simulink model "Diagrama2"  (R2023b)
settings: Solver=VariableStepAuto  StartTime=0.0  StopTime=10.0  RelTol=1e-3
settings Model: Creator=Roberd  LastModifiedBy=Roberd

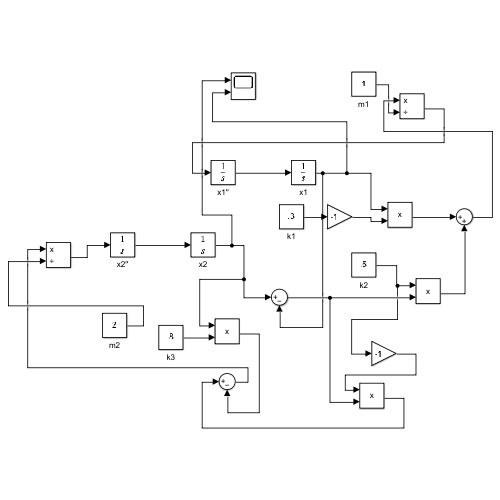
[thumbnail: Simulink's stored preview of the top-level diagram]
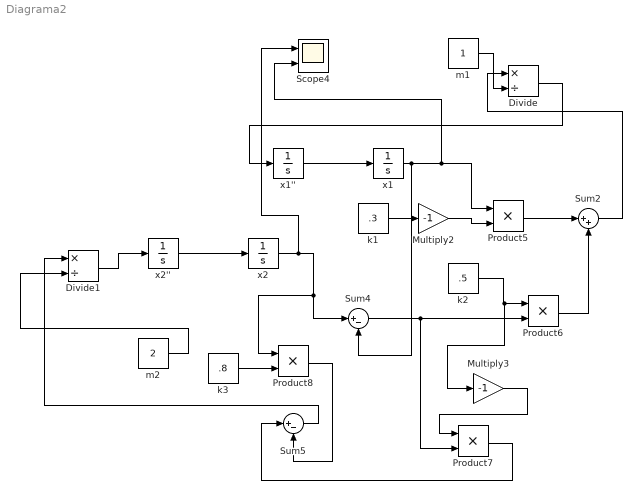
== system Diagrama2 ==
  Divide : Product  Inputs=*/
  Divide1 : Product  Inputs=*/
  Multiply2 : Gain  Gain=-1
  Multiply3 : Gain  Gain=-1
  Product{5..8} (4 alike) : Product
  Scope4 : Scope  NumInputPorts=2
  Sum2 : Sum  Inputs=|++
  Sum4 : Sum  Inputs=|+-
  Sum5 : Sum  Inputs=|+-
  k1 : Constant  Value=.3
  k2 : Constant  Value=.5
  k3 : Constant  Value=.8
  m1 : Constant
  m2 : Constant  Value=2
  x1 : Integrator
  x1'' : Integrator  InitialCondition=1
  x2 : Integrator
  x2'' : Integrator
  wires:
  Product7/1 -> Sum5/1
  m2/1 -> Divide1/2
  x1''/1 -> x1/1
  x2''/1 -> x2/1
  Sum2/1 -> Divide/1
  Product8/1 -> Sum5/2
  Multiply3/1 -> Product7/1
  Sum5/1 -> Divide1/1
  k3/1 -> Product8/2
  Divide1/1 -> x2''/1
  m1/1 -> Divide/2
  Sum4/1 -> Product7/2, Product6/2
  k1/1 -> Multiply2/1
  Product6/1 -> Sum2/2
  x2/1 -> Scope4/1, Product8/1, Sum4/1
  k2/1 -> Multiply3/1, Product6/1
  Divide/1 -> x1''/1
  Multiply2/1 -> Product5/2
  x1/1 -> Scope4/2, Product5/1, Sum4/2
  Product5/1 -> Sum2/1
